simulink model "DQAvgInvEquivalentFOCModel2019"  (R2019a)
settings: Solver=FixedStepAuto  StartTime=0.0  StopTime=3184  FixedStep=2.5e-5  RelTol=1e-3
InitFcn:
  | run('PowerTrainParams.m')
values from neighbouring files (symbols this model uses):
  A = V_full - V_exp    (= 0.45)    [PowerTrainParams.m]
  B = 1/C_exp    (= 0.000185185185185)    [PowerTrainParams.m]
  B_f = 0.0025    [PowerTrainParams.m]
  E_0 = V_exp    (= 3.7)    [PowerTrainParams.m]
  G_r = 0.75    [PowerTrainParams.m]
  J = 0.0922    [PowerTrainParams.m]
  K = (V_exp - V_nom)*(C_max - C_nom)/(C_max*C_nom)    (= 2.19298245614e-06)    [PowerTrainParams.m]
  Ki_I = 100    [PowerTrainParams.m]
  Ki_T = 1    [PowerTrainParams.m]
  Kp_I = 1    [PowerTrainParams.m]
  Kp_T = 1    [PowerTrainParams.m]
  L_d = 0.000126    [PowerTrainParams.m]
  L_q = 0.000118    [PowerTrainParams.m]
  lambda = 0.0664    [PowerTrainParams.m]
  n_climb = 2092    [PowerTrainParams.m]
  n_cruise = 1291    [PowerTrainParams.m]
  n_glide = 1291    [PowerTrainParams.m]
  n_land = 4929    [PowerTrainParams.m]
  N_par = 6    [PowerTrainParams.m]
  N_ser = 176    [PowerTrainParams.m]
  n_takeoff = 4929    [PowerTrainParams.m]
  p = 10    [PowerTrainParams.m]
  Q = C_max    (= 10260)    [PowerTrainParams.m]
  q = 3    [PowerTrainParams.m]
  R_int = 0.004    [PowerTrainParams.m]
  R_s = 0.0105    [PowerTrainParams.m]
  t_change = 5    [PowerTrainParams.m]
  t_climb = 44+t_change    (= 49)    [PowerTrainParams.m]
  T_climb = 42.94    [PowerTrainParams.m]
  t_cruise = 2875+t_change    (= 2880)    [PowerTrainParams.m]
  T_cruise = 19.1    [PowerTrainParams.m]
  t_glide = 105+t_change    (= 110)    [PowerTrainParams.m]
  T_glide = 17.2    [PowerTrainParams.m]
  t_land = 100+t_change    (= 105)    [PowerTrainParams.m]
  T_land = 238    [PowerTrainParams.m]
  t_takeoff = 30+t_change    (= 35)    [PowerTrainParams.m]
  T_takeoff = 238    [PowerTrainParams.m]
  V_dc = 3.7*N_ser    (= 651.2)    [PowerTrainParams.m]
libraries: simulink x27, eeGeneralControl x3, eeTransforms x2, spsTriangleGeneratorLib x1
settings Model: Creator=trgre  LastModifiedBy=Tim Zhao
settings DataIOCC: SaveTime=off
settings SimscapeCC: EditingMode=Restricted

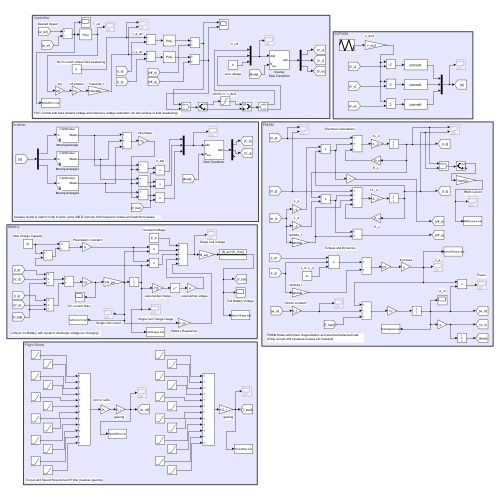
[thumbnail: Simulink's stored preview of the top-level diagram]
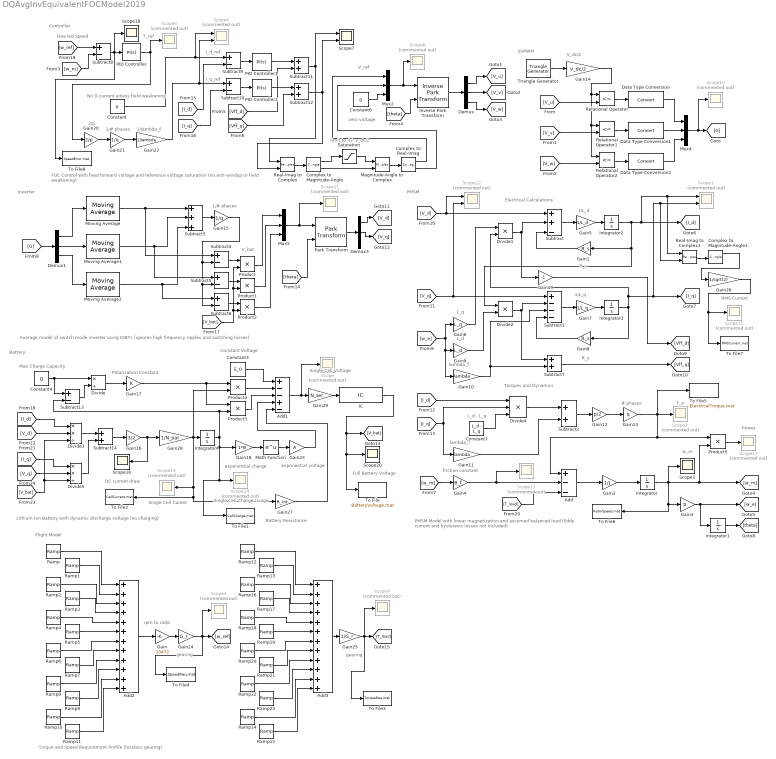
== system DQAvgInvEquivalentFOCModel2019 ==
  note: gearing
  note: Full Battery Voltage
  note: Single Cell Voltage
  note: Single Cell Curent
  note: limit to +/- v_dc/2
  note: w_m
  note: Power
  note: RMS Current
  note: Battery Resistance
  note: Single Cell Charge Usage
  note: DC current draw
  note: gearing
  note: Torque and Speed Requirement Profile (lossless gearing)
  note: rpm to rad/s
  note: Flight Model
  note: exponential voltage
  note: exponential charge
  note: Polarization Constant
  note: Max Charge Capacity
  note: Constant Voltage
  note: Lithium Ion Battery with dynamic discharge voltage (no charging)
  note: Battery
  note: V_ref
  note: I_q_ref
  note: I_d_ref
  note: No D current unless field weakening
  note: 1/lambda_f
  note: T_ref
  note: FOC Control with feed forward voltage and reference voltage saturation (no anti-windup or field weakening)
  note: T_e
  note: V_bat
  note: 1/# phases
  note: Average model of switch mode inverter using IGBTs (ignores high frequency ripples and switching losses)
  note: # phases
  note: L_d - L_q
  note: lambda_f
  note: L_d
  note: 1/L_q
  note: L_q
  note: R_s
  note: 1/L_d
  note: friction constant
  note: Inverter
  note: PMSM
  note: Torques and Dynamics
  note: Electrical Calculations
  note: PMSM Model with linear magnetization and assumed balanced load
      | (Eddy current and hysteresis losses not included)
  note: Controller
  note: SVPWM
  note: Desired Speed
  note: zero voltage
  note: V_dc/2
  note: R_s
  note: lambda_f
  note: 2/p
  note: 1/# phases
  Add : Sum  Inputs=+--
  Add1 : Sum  Inputs=+--+-
  Add2 : Sum  Inputs=++++++++++++
  Add3 : Sum  Inputs=++++++++++++
  Complex to Magnitude-Angle : ComplexToMagnitudeAngle
  Complex to Magnitude-Angle1 : ComplexToMagnitudeAngle
  Complex to Real-Imag : ComplexToRealImag
  Constant : Constant  Value=0
  Constant3 : Constant  Value=E_0
  Constant4 : Constant  Value=Q
  Constant6 : Constant  Value=0
  Constant7 : Constant  Value=L_d - L_q
  Data Type Conversion : DataTypeConversion
  Data Type Conversion1 : DataTypeConversion
  Data Type Conversion2 : DataTypeConversion
  Demux : Demux  Outputs=3
  Demux1 : Demux  Outputs=3
  Demux3 : Demux  Outputs=3
  Divide : Product  Inputs=*/
  Divide1 : Product  Inputs=**
  Divide2 : Product  Inputs=**
  Divide3 : Product  Inputs=**/
  Divide4 : Product  Inputs=***
  Divide5 : Product  Inputs=**/
  Gain : Gain  Gain=.10472
  Gain1 : Gain  Gain=R_s
  Gain10 : Gain  Gain=lambda
  Gain11 : Gain  Gain=lambda
  Gain12 : Gain  Gain=p/2
  Gain13 : Gain  Gain=q
  Gain14 : Gain  Gain=V_dc/2
  Gain15 : Gain  Gain=1/q
  Gain16 : Gain  Gain=3/2
  Gain17 : Gain  Gain=K
  Gain18 : Gain  Gain=-1*B
  Gain19 : Gain  Gain=-1
  Gain2 : Gain  Gain=1/J
  Gain20 : Gain  Gain=2/p
  Gain21 : Gain  Gain=1/q
  Gain22 : Gain  Gain=1/lambda
  Gain23 : Gain  Gain=A
  Gain24 : Gain  Gain=G_r
  Gain25 : Gain  Gain=1/G_r
  Gain26 : Gain  Gain=1/sqrt(2)
  Gain27 : Gain  Gain=R_int
  Gain28 : Gain  Gain=1/N_par
  Gain29 : Gain  Gain=N_ser
  Gain3 : Gain  Gain=p
  Gain4 : Gain  Gain=B_f
  Gain5 : Gain  Gain=1/L_d
  Gain6 : Gain  Gain=L_q
  Gain7 : Gain  Gain=1/L_q
  Gain8 : Gain  Gain=R_s
  Gain9 : Gain  Gain=L_d
  IC : InitialCondition  Value=N_ser*(E_0+A)
  Integrator{,1..4} (5 alike) : Integrator
  Inverse Park Transform : eeTransforms/Inverse Park Transform  AxisAlignment=Q-axis  PowerInvariant=off
  Magnitude-Angle to Complex : MagnitudeAngleToComplex
  Math Function : Math  SaturateOnIntegerOverflow=on
  Moving Average : eeGeneralControl/Moving Average  VariantControl=Variant1  LabelModeActiveChoice=Continuous  f=5000  x0=0  BufferSize=8192  Ts=0
      settings: SourceProductBaseCode=PS
  Moving Average1 : eeGeneralControl/Moving Average  VariantControl=Variant1  LabelModeActiveChoice=Continuous  f=5000  x0=0  BufferSize=8192  Ts=0
      settings: SourceProductBaseCode=PS
  Moving Average2 : eeGeneralControl/Moving Average  VariantControl=Variant1  LabelModeActiveChoice=Continuous  f=5000  x0=0  BufferSize=8192  Ts=0
      settings: SourceProductBaseCode=PS
  Mux2 : Mux  Inputs=3
  Mux4 : Mux  Inputs=3
  Mux5 : Mux  Inputs=3
  PID Controller : simulink/Continuous/PID Controller  Controller=PI  Form=Parallel  TimeDomain=Continuous-time  SampleTime=-1  IntegratorMethod=Forward Euler  FilterMethod=Forward Euler  ControllerParametersSource=internal  P=Kp_T  I=Ki_T  D=0  UseFilter=on  N=100  TunerSelectOption=Transfer Function Based (PID Tuner App)  InitialConditionSource=internal  InitialConditionForIntegrator=0  InitialConditionForFilter=0  DifferentiatorICPrevScaledInput=0  ExternalReset=none  TrackingMode=off  Kt=1  LimitOutput=off  UpperSaturationLimit=inf  LowerSaturationLimit=-inf  LinearizeAsGain=on  AntiWindupMode=none  Kb=1  POutMin=[]  POutMax=[]  IOutMin=[]  IOutMax=[]  DOutMin=[]  DOutMax=[]  NOutMin=[]  NOutMax=[]  SumOutMin=[]  SumOutMax=[]  SaturationOutMin=[]  SaturationOutMax=[]  PParamMin=[]  PParamMax=[]  IParamMin=[]  IParamMax=[]  DParamMin=[]  DParamMax=[]  NParamMin=[]  NParamMax=[]  KbParamMin=[]  KbParamMax=[]  KtParamMin=[]  KtParamMax=[]  KbOutMin=[]  KbOutMax=[]  KtOutMin=[]  KtOutMax=[]  IntegratorOutMin=[]  IntegratorOutMax=[]  FilterOutMin=[]  FilterOutMax=[]  SumI1OutMin=[]  SumI1OutMax=[]  SumI2OutMin=[]  SumI2OutMax=[]  SumI3OutMin=[]  SumI3OutMax=[]  SumI4OutMin=[]  SumI4OutMax=[]  SumDOutMin=[]  SumDOutMax=[]  DifferentiatorOutMin=[]  DifferentiatorOutMax=[]  FilterDiffOutCoefMin=[]  FilterDiffOutCoefMax=[]  ReciprocalOutMin=[]  ReciprocalOutMax=[]  SumDenOutMin=[]  SumDenOutMax=[]  SumNumOutMin=[]  SumNumOutMax=[]  DivideOutMin=[]  DivideOutMax=[]  IntegratorContinuousStateAttributes=''  IntegratorStateMustResolveToSignalObject=off  IntegratorRTWStateStorageClass=Auto  FilterContinuousStateAttributes=''  FilterStateMustResolveToSignalObject=off  FilterRTWStateStorageClass=Auto  ParallelPVariant=InternalParameters  IdealPVariant=Disabled  IVariant=InternalParameters  DVariant=Disabled  IntegratorVariant=Continuous  SatVariant=Disabled  AWVariant=Passthrough  PCopyVariant=Disabled  TRVariant=Disabled  FdbkBlocksVariant=Forward  IdealPFdbkVariant=Disabled  SatFdbkVariant=Disabled  DerivativeFilterVariant=Disabled  NVariant=Disabled  NCopyVariant=Disabled_SignalSpec  FilterICVariant=Disabled  IntegratorICVariant=InternalICs  ExternalResetVariant=Disabled  TRSumVariant=Passthrough  SumFdbkVariant=Disabled  SumVariant=Sum_PI
  PID Controller1 : simulink/Continuous/PID Controller  Controller=PI  Form=Parallel  TimeDomain=Continuous-time  SampleTime=-1  IntegratorMethod=Forward Euler  FilterMethod=Forward Euler  ControllerParametersSource=internal  P=Kp_I  I=Ki_I  D=0  UseFilter=on  N=100  TunerSelectOption=Transfer Function Based (PID Tuner App)  InitialConditionSource=internal  InitialConditionForIntegrator=0  InitialConditionForFilter=0  DifferentiatorICPrevScaledInput=0  ExternalReset=none  TrackingMode=off  Kt=1  LimitOutput=off  UpperSaturationLimit=inf  LowerSaturationLimit=-inf  LinearizeAsGain=on  AntiWindupMode=none  Kb=1  POutMin=[]  POutMax=[]  IOutMin=[]  IOutMax=[]  DOutMin=[]  DOutMax=[]  NOutMin=[]  NOutMax=[]  SumOutMin=[]  SumOutMax=[]  SaturationOutMin=[]  SaturationOutMax=[]  PParamMin=[]  PParamMax=[]  IParamMin=[]  IParamMax=[]  DParamMin=[]  DParamMax=[]  NParamMin=[]  NParamMax=[]  KbParamMin=[]  KbParamMax=[]  KtParamMin=[]  KtParamMax=[]  KbOutMin=[]  KbOutMax=[]  KtOutMin=[]  KtOutMax=[]  IntegratorOutMin=[]  IntegratorOutMax=[]  FilterOutMin=[]  FilterOutMax=[]  SumI1OutMin=[]  SumI1OutMax=[]  SumI2OutMin=[]  SumI2OutMax=[]  SumI3OutMin=[]  SumI3OutMax=[]  SumI4OutMin=[]  SumI4OutMax=[]  SumDOutMin=[]  SumDOutMax=[]  DifferentiatorOutMin=[]  DifferentiatorOutMax=[]  FilterDiffOutCoefMin=[]  FilterDiffOutCoefMax=[]  ReciprocalOutMin=[]  ReciprocalOutMax=[]  SumDenOutMin=[]  SumDenOutMax=[]  SumNumOutMin=[]  SumNumOutMax=[]  DivideOutMin=[]  DivideOutMax=[]  IntegratorContinuousStateAttributes=''  IntegratorStateMustResolveToSignalObject=off  IntegratorRTWStateStorageClass=Auto  FilterContinuousStateAttributes=''  FilterStateMustResolveToSignalObject=off  FilterRTWStateStorageClass=Auto  ParallelPVariant=InternalParameters  IdealPVariant=Disabled  IVariant=InternalParameters  DVariant=Disabled  IntegratorVariant=Continuous  SatVariant=Disabled  AWVariant=Passthrough  PCopyVariant=Disabled  TRVariant=Disabled  FdbkBlocksVariant=Forward  IdealPFdbkVariant=Disabled  SatFdbkVariant=Disabled  DerivativeFilterVariant=Disabled  NVariant=Disabled  NCopyVariant=Disabled_SignalSpec  FilterICVariant=Disabled  IntegratorICVariant=InternalICs  ExternalResetVariant=Disabled  TRSumVariant=Passthrough  SumFdbkVariant=Disabled  SumVariant=Sum_PI
  PID Controller2 : simulink/Continuous/PID Controller  Controller=PI  Form=Parallel  TimeDomain=Continuous-time  SampleTime=-1  IntegratorMethod=Forward Euler  FilterMethod=Forward Euler  ControllerParametersSource=internal  P=Kp_I  I=Ki_I  D=0  UseFilter=on  N=100  TunerSelectOption=Transfer Function Based (PID Tuner App)  InitialConditionSource=internal  InitialConditionForIntegrator=0  InitialConditionForFilter=0  DifferentiatorICPrevScaledInput=0  ExternalReset=none  TrackingMode=off  Kt=1  LimitOutput=off  UpperSaturationLimit=inf  LowerSaturationLimit=-inf  LinearizeAsGain=on  AntiWindupMode=none  Kb=1  POutMin=[]  POutMax=[]  IOutMin=[]  IOutMax=[]  DOutMin=[]  DOutMax=[]  NOutMin=[]  NOutMax=[]  SumOutMin=[]  SumOutMax=[]  SaturationOutMin=[]  SaturationOutMax=[]  PParamMin=[]  PParamMax=[]  IParamMin=[]  IParamMax=[]  DParamMin=[]  DParamMax=[]  NParamMin=[]  NParamMax=[]  KbParamMin=[]  KbParamMax=[]  KtParamMin=[]  KtParamMax=[]  KbOutMin=[]  KbOutMax=[]  KtOutMin=[]  KtOutMax=[]  IntegratorOutMin=[]  IntegratorOutMax=[]  FilterOutMin=[]  FilterOutMax=[]  SumI1OutMin=[]  SumI1OutMax=[]  SumI2OutMin=[]  SumI2OutMax=[]  SumI3OutMin=[]  SumI3OutMax=[]  SumI4OutMin=[]  SumI4OutMax=[]  SumDOutMin=[]  SumDOutMax=[]  DifferentiatorOutMin=[]  DifferentiatorOutMax=[]  FilterDiffOutCoefMin=[]  FilterDiffOutCoefMax=[]  ReciprocalOutMin=[]  ReciprocalOutMax=[]  SumDenOutMin=[]  SumDenOutMax=[]  SumNumOutMin=[]  SumNumOutMax=[]  DivideOutMin=[]  DivideOutMax=[]  IntegratorContinuousStateAttributes=''  IntegratorStateMustResolveToSignalObject=off  IntegratorRTWStateStorageClass=Auto  FilterContinuousStateAttributes=''  FilterStateMustResolveToSignalObject=off  FilterRTWStateStorageClass=Auto  ParallelPVariant=InternalParameters  IdealPVariant=Disabled  IVariant=InternalParameters  DVariant=Disabled  IntegratorVariant=Continuous  SatVariant=Disabled  AWVariant=Passthrough  PCopyVariant=Disabled  TRVariant=Disabled  FdbkBlocksVariant=Forward  IdealPFdbkVariant=Disabled  SatFdbkVariant=Disabled  DerivativeFilterVariant=Disabled  NVariant=Disabled  NCopyVariant=Disabled_SignalSpec  FilterICVariant=Disabled  IntegratorICVariant=InternalICs  ExternalResetVariant=Disabled  TRSumVariant=Passthrough  SumFdbkVariant=Disabled  SumVariant=Sum_PI
  Park Transform : eeTransforms/Park Transform  AxisAlignment=Q-axis  PowerInvariant=off
  Product{,1..5} (6 alike) : Product
  Ramp : simulink/Sources/Ramp  slope=n_takeoff/t_change  start=0  InitialOutput=0
  Ramp1 : simulink/Sources/Ramp  slope=-1*n_takeoff/t_change  start=t_change  InitialOutput=0
  Ramp10 : simulink/Sources/Ramp  slope=-1*n_land/t_change  start=t_takeoff+t_climb+t_cruise+t_glide+t_land  InitialOutput=0
  Ramp11 : simulink/Sources/Ramp  slope=n_land/t_change  start=t_takeoff+t_climb+t_cruise+t_glide+t_land+t_change  InitialOutput=0
  Ramp12 : simulink/Sources/Ramp  slope=T_takeoff/t_change  start=0  InitialOutput=0
  Ramp13 : simulink/Sources/Ramp  slope=-1*T_takeoff/t_change  start=t_change  InitialOutput=0
  Ramp14 : simulink/Sources/Ramp  slope=-1*T_land/t_change  start=t_takeoff+t_climb+t_cruise+t_glide+t_land  InitialOutput=0
  Ramp15 : simulink/Sources/Ramp  slope=T_land/t_change  start=t_takeoff+t_climb+t_cruise+t_glide+t_land+t_change  InitialOutput=0
  Ramp16 : simulink/Sources/Ramp  slope=(T_climb-T_takeoff)/t_change  start=t_takeoff  InitialOutput=0
  Ramp17 : simulink/Sources/Ramp  slope=-1*(T_climb-T_takeoff)/t_change  start=t_takeoff+t_change  InitialOutput=0
  Ramp18 : simulink/Sources/Ramp  slope=(T_cruise-T_climb)/t_change  start=t_takeoff+t_climb  InitialOutput=0
  Ramp19 : simulink/Sources/Ramp  slope=-1*(T_cruise-T_climb)/t_change  start=t_takeoff+t_climb+t_change  InitialOutput=0
  Ramp2 : simulink/Sources/Ramp  slope=(n_climb-n_takeoff)/t_change  start=t_takeoff  InitialOutput=0
  Ramp20 : simulink/Sources/Ramp  slope=(T_glide-T_cruise)/t_change  start=t_takeoff+t_climb+t_cruise  InitialOutput=0
  Ramp21 : simulink/Sources/Ramp  slope=-1*(T_glide-T_cruise)/t_change  start=t_takeoff+t_climb+t_cruise+t_change  InitialOutput=0
  Ramp22 : simulink/Sources/Ramp  slope=(T_land-T_glide)/t_change  start=t_takeoff+t_climb+t_cruise+t_glide  InitialOutput=0
  Ramp23 : simulink/Sources/Ramp  slope=-1*(T_land-T_glide)/t_change  start=t_takeoff+t_climb+t_cruise+t_glide+t_change  InitialOutput=0
  Ramp3 : simulink/Sources/Ramp  slope=-1*(n_climb-n_takeoff)/t_change  start=t_takeoff+t_change  InitialOutput=0
  Ramp4 : simulink/Sources/Ramp  slope=(n_cruise-n_climb)/t_change  start=t_takeoff+t_climb  InitialOutput=0
  Ramp5 : simulink/Sources/Ramp  slope=-1*(n_cruise-n_climb)/t_change  start=t_takeoff+t_climb+t_change  InitialOutput=0
  Ramp6 : simulink/Sources/Ramp  slope=(n_glide-n_cruise)/t_change  start=t_takeoff+t_climb+t_cruise  InitialOutput=0
  Ramp7 : simulink/Sources/Ramp  slope=-1*(n_glide-n_cruise)/t_change  start=t_takeoff+t_climb+t_cruise+t_change  InitialOutput=0
  Ramp8 : simulink/Sources/Ramp  slope=(n_land-n_glide)/t_change  start=t_takeoff+t_climb+t_cruise+t_glide  InitialOutput=0
  Ramp9 : simulink/Sources/Ramp  slope=-1*(n_land-n_glide)/t_change  start=t_takeoff+t_climb+t_cruise+t_glide+t_change  InitialOutput=0
  Real-Imag to Complex : RealImagToComplex
  Real-Imag to Complex1 : RealImagToComplex
  Relational Operator : RelationalOperator  Operator=<=  OutDataTypeStr=boolean  RndMeth=Simplest
  Relational Operator1 : RelationalOperator  Operator=<=  OutDataTypeStr=boolean  RndMeth=Simplest
  Relational Operator2 : RelationalOperator  Operator=<=  OutDataTypeStr=boolean  RndMeth=Simplest
  Saturation : Saturate  UpperLimit=V_dc/2  LowerLimit=-1*V_dc/2
  Scope{,2,4..5,8..11,13..15,17,19} (13 alike) : Scope  Commented=on
  Scope1 : Scope  Commented=on  NumInputPorts=2
  Scope12 : Scope  Commented=on  NumInputPorts=2
  Scope{3,16,18,20} (4 alike) : Scope
  Scope6 : Scope  Commented=on  NumInputPorts=2
  Scope7 : Scope  NumInputPorts=2
  Subtract : Sum  Inputs=++-
  Subtract1 : Sum  Inputs=+---
  Subtract{4..6,8..10,13} (7 alike) : Sum  Inputs=+-
  Subtract{2,7,11..12,14} (5 alike) : Sum
  Subtract3 : Sum  Inputs=+++
  To File : ToFile  Filename=BatteryVoltage.mat  SaveFormat=Timeseries
  To File1 : ToFile  Filename=CellCharge.mat  SaveFormat=Timeseries
  To File2 : ToFile  Filename=CellCurrent.mat  SaveFormat=Timeseries
  To File3 : ToFile  Filename=TorqueReq.mat  SaveFormat=Timeseries
  To File4 : ToFile  Filename=SpeedReq.mat  SaveFormat=Timeseries
  To File5 : ToFile  Filename=ElectricalTorque.mat  SaveFormat=Timeseries
  To File6 : ToFile  Filename=RotorSpeed.mat  SaveFormat=Timeseries
  To File7 : ToFile  Filename=RMSCurrent.mat  SaveFormat=Timeseries
  To File8 : ToFile  Filename=SpeedError.mat  SaveFormat=Timeseries
  Triangle Generator : spsTriangleGeneratorLib/Triangle Generator  Freq=5000  Phase=90  Ts=0
  wires:
  Inverse Park Transform/1 -> Demux/1
  Gain14/1 -> Relational Operator/1, Relational Operator1/1, Relational Operator2/1
  Mux2/1 -> Scope8/1, Inverse Park Transform/1
  Constant6/1 -> Mux2/3
  [V_u] -> Relational Operator/2
  [V_v] -> Relational Operator1/2
  [V_w] -> Relational Operator2/2
  Demux/1 -> [V_u]
  Demux/2 -> [V_v]
  Demux/3 -> [V_w]
  [G] -> Demux1/1
  [V_d] -> Scope12/1, Subtract/1
  Add/1 -> Gain2/1
  Gain2/1 -> Integrator/1
  Integrator/1 -> To File6/1, Gain3/1, Product5/2, [w_m], Scope3/1
  Gain3/1 -> Integrator1/1, [w_e]
  [theta] -> Inverse Park Transform/2
  [w_m] -> Gain4/1
  Gain4/1 -> Scope13/1, Add/2
  Integrator1/1 -> [theta]
  Subtract/1 -> Gain5/1
  Gain1/1 -> Subtract/3
  [w_e] -> Gain10/1, Gain9/1, Gain6/1
  Divide1/1 -> Gain19/1, Subtract/2
  Gain6/1 -> Divide1/1
  [V_q] -> Scope12/2, Subtract1/1
  Subtract1/1 -> Gain7/1
  Gain5/1 -> Integrator2/1
  Integrator2/1 -> Scope1/1, Real-Imag to Complex1/1, [I_d], Divide2/1, Gain1/1
  Gain7/1 -> Integrator3/1
  Integrator3/1 -> Divide1/2, Real-Imag to Complex1/2, Scope1/2, [I_q], Gain8/1
  Gain8/1 -> Subtract1/4
  Gain9/1 -> Divide2/2
  Divide2/1 -> Subtract7/1, Subtract1/2
  Gain10/1 -> Subtract7/2, Subtract1/3
  [I_q] -> Gain11/1, Divide4/2
  [I_d] -> Divide4/1
  Constant7/1 -> Divide4/3
  Gain11/1 -> Subtract2/2
  Divide4/1 -> Subtract2/1
  Subtract2/1 -> Gain12/1
  Gain12/1 -> Gain13/1
  Triangle Generator/1 -> Gain14/1
  Mux4/1 -> Scope10/1, [G]
  Demux1/2 -> Moving Average1/1
  Demux1/1 -> Moving Average/1
  Demux1/3 -> Moving Average2/1
  Subtract3/1 -> Gain15/1
  Moving Average/1 -> Subtract3/1, Subtract4/1
  Moving Average1/1 -> Subtract5/1, Subtract3/2
  Moving Average2/1 -> Subtract6/1, Subtract3/3
  Gain15/1 -> Subtract6/2, Subtract5/2, Subtract4/2
  Subtract4/1 -> Product/1
  Subtract6/1 -> Product2/1
  Subtract5/1 -> Product1/1
  Mux5/1 -> Scope11/1, Park Transform/1
  [theta] -> Park Transform/2
  Park Transform/1 -> Demux3/1
  Demux3/1 -> [V_d]
  Demux3/2 -> [V_q]
  Relational Operator/1 -> Data Type Conversion/1
  Relational Operator1/1 -> Data Type Conversion1/1
  Relational Operator2/1 -> Data Type Conversion2/1
  Data Type Conversion2/1 -> Mux4/3
  Data Type Conversion1/1 -> Mux4/2
  Data Type Conversion/1 -> Mux4/1
  [w_ref] -> Subtract8/1
  [w_m] -> Subtract8/2
  [I_d] -> Subtract9/2
  [I_q] -> Subtract10/2
  Subtract8/1 -> To File8/1, Scope18/1, PID Controller/1
  PID Controller/1 -> Gain20/1, Scope5/1
  Subtract9/1 -> PID Controller1/1
  Subtract10/1 -> PID Controller2/1
  Gain19/1 -> [Vff_d]
  Subtract7/1 -> [Vff_q]
  Gain20/1 -> Gain21/1
  Gain21/1 -> Gain22/1
  Constant/1 -> Subtract9/1, Scope6/1
  Gain22/1 -> Subtract10/1, Scope6/2
  Magnitude-Angle to Complex/1 -> Complex to Real-Imag/1
  Real-Imag to Complex/1 -> Complex to Magnitude-Angle/1
  Complex to Magnitude-Angle/2 -> Magnitude-Angle to Complex/2
  Saturation/1 -> Magnitude-Angle to Complex/1
  Complex to Magnitude-Angle/1 -> Saturation/1
  Complex to Real-Imag/1 -> Mux2/1
  Complex to Real-Imag/2 -> Mux2/2
  Product/1 -> Mux5/1
  Product1/1 -> Mux5/2
  Product2/1 -> Mux5/3
  [V_bat] -> Product2/2, Product1/2, Product/2
  Constant3/1 -> Add1/1
  Constant4/1 -> Divide/1, Subtract13/1
  Subtract13/1 -> Divide/2
  Divide/1 -> Gain17/1
  Gain17/1 -> Product3/1, Product4/1
  Gain18/1 -> Math Function/1
  Math Function/1 -> Gain23/1
  Add1/1 -> Scope/1, Gain29/1
  [T_load] -> Add/3
  Ramp5/1 -> Add2/6
  Ramp4/1 -> Add2/5
  Ramp3/1 -> Add2/4
  Ramp2/1 -> Add2/3
  Ramp1/1 -> Add2/2
  Ramp/1 -> Add2/1
  Ramp6/1 -> Add2/7
  Ramp7/1 -> Add2/8
  Ramp8/1 -> Add2/9
  Ramp9/1 -> Add2/10
  Ramp10/1 -> Add2/11
  Ramp11/1 -> Add2/12
  Ramp19/1 -> Add3/6
  Ramp21/1 -> Add3/8
  Ramp23/1 -> Add3/10
  Ramp18/1 -> Add3/5
  Ramp13/1 -> Add3/2
  Ramp14/1 -> Add3/11
  Ramp16/1 -> Add3/3
  Ramp17/1 -> Add3/4
  Ramp12/1 -> Add3/1
  Ramp22/1 -> Add3/9
  Ramp20/1 -> Add3/7
  Ramp15/1 -> Add3/12
  Add2/1 -> Gain/1
  Gain25/1 -> To File3/1, Scope9/1, [T_load]
  Add3/1 -> Gain25/1
  [I_d] -> Divide3/1
  [V_d] -> Divide3/2
  [V_q] -> Divide5/2
  [I_q] -> Divide5/1
  [V_bat] -> Divide3/3, Divide5/3
  Divide3/1 -> Subtract14/1
  Divide5/1 -> Subtract14/2
  Gain16/1 -> Gain28/1, Scope16/1
  Subtract14/1 -> Gain16/1
  Real-Imag to Complex1/1 -> Complex to Magnitude-Angle1/1
  Complex to Magnitude-Angle1/1 -> Gain26/1
  Gain26/1 -> To File7/1, Scope15/1
  Product5/1 -> Scope17/1
  PID Controller2/1 -> Subtract12/1
  PID Controller1/1 -> Subtract11/1
  Subtract11/1 -> Real-Imag to Complex/1, Scope7/1
  Subtract12/1 -> Real-Imag to Complex/2, Scope7/2
  [Vff_d] -> Subtract11/2
  [Vff_q] -> Subtract12/2
  Integrator4/1 -> To File1/1, Scope14/1, Gain18/1, Product3/2, Subtract13/2
  Product4/1 -> Add1/2
  Gain28/1 -> Product4/2, To File2/1, Gain27/1, Scope19/1, Integrator4/1
  Gain27/1 -> Add1/5
  Gain23/1 -> Add1/4
  Product3/1 -> Add1/3
  Gain29/1 -> IC/1
  Gain13/1 -> Scope2/1, Product5/1, Add/1, To File5/1
  Gain24/1 -> To File4/1, Scope4/1, [w_ref]
  Gain/1 -> Gain24/1
  IC/1 -> [V_bat], To File/1, Scope20/1
